simulink model "EENG650assignment2_V_2"  (R2020b)
settings: Solver=VariableStepAuto  StartTime=0.0  StopTime=10.0  RelTol=1e-3
settings Model: EnablePacing=on  Creator=Kelvin  LastModifiedBy=Kelvin

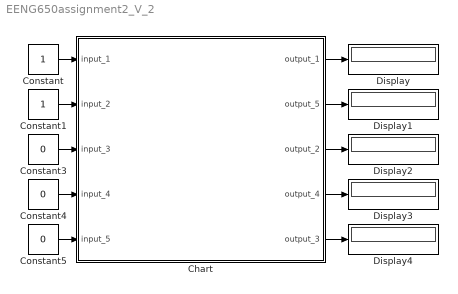
== system EENG650assignment2_V_2 ==
  Chart : Stateflow chart  TreatAsAtomicUnit=on
  Constant : Constant
  Constant1 : Constant
  Constant3 : Constant  Value=0
  Constant4 : Constant  Value=0
  Constant5 : Constant  Value=0
  Display{,1..4} (5 alike) : Display
  wires:
  Constant/1 -> Chart/1(input_1)
  Constant1/1 -> Chart/2(input_2)
  Constant3/1 -> Chart/3(input_3)
  Constant4/1 -> Chart/4(input_4)
  Constant5/1 -> Chart/5(input_5)
  Chart/1(output_1) -> Display/1
  Chart/2(output_5) -> Display1/1
  Chart/3(output_2) -> Display2/1
  Chart/4(output_4) -> Display3/1
  Chart/5(output_3) -> Display4/1

== stateflow chart EENG650assignment2_V_2/Chart ==
  state State1
    entry:
    output_1 = input_1;
  state State0
  state State2
    entry:
    output_2 = input_2;
  state Sate8
    entry:
    output_3 = input_3;
  note: return hand-set
  note: END
  note: Start
  note: Wait
  note: Talk
  note: Talking
  state State6
    entry:
    output_5 = input_5;
  state Sate4
    entry:
    output_4 = input_1;
  note: Record
  note: Play message
  Sate8 -> State0 [order 1] : [input_3 ==1]
  (default) -> State0
  State2 -> State2 [order 2] : [ input_2==0]
  State1 -> State2 [order 1] : [input_1 ==1]
  State2 -> Sate8 [order 1] : [input_2==1]
  State0 -> State1
  Sate8 -> (junction 69) [order 2]
  State6 -> State0 [order 1] : [input_5==1]
  Sate4 -> State0 [order 2] : [input_4 ==0]
  State1 -> Sate4 [order 2] : [input_1 ==0]
  State6 -> (junction 69) [order 2]
  Sate4 -> State6 [order 1] : [input_4 ==1]
  data: input_1 input; input_2 input; output_1 output; output_5 output; output_2 output; output_4 output; input_3 input; input_4 input; input_5 input; output_3 output
